simulink model "HinfDesign1_closed"  (R2018b)
settings: Solver=VariableStepAuto  StartTime=0.0  StopTime=200  RelTol=1e-3
model workspace: external: MATLAB File C:\Users\Yavuz\Documents\MATLAB\constants.m (data not in the file)
values from neighbouring files (symbols this model uses):
  alpha = 0.5736    [constants.m]
  c_damp = 0.00495    [constants.m]
  delay = 0.8    [constants.m]
  dis_torque = 0.001    [constants.m]
  in_nu = 0.0001    [constants.m]
  J_r = 0.0004    [constants.m]
  J_s = 31.38    [constants.m]
  noise = 10^-9    (= 1e-09)    [constants.m]
  T_sat = 0.05    [constants.m]
  time_cons = 0.5    [constants.m]
  w_mode = 2.6268    [constants.m]
  w_sat = 2800*2*pi/60    (= 293.215314335)    [constants.m]
libraries: cstblocks x1
settings Model: Creator=Yavuz  LastModifiedBy=Yavuz
settings DebuggingCC: AlgebraicLoopMsg=none

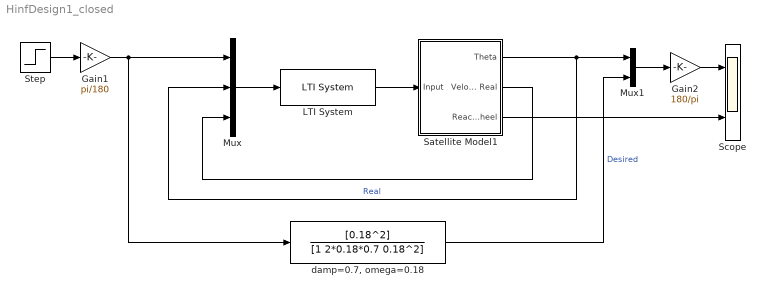
== system HinfDesign1_closed ==
  Gain1 : Gain  Gain=pi/180
  Gain2 : Gain  Gain=180/pi
  LTI System : cstblocks/LTI System  sys=K  IC=[]
  Mux : Mux  Inputs=3
  Mux1 : Mux  Inputs=2
  Satellite Model1 : Subsystem
  Scope : Scope  NumInputPorts=2
  Step : Step  Time=0  After=2.5  SampleTime=0
  "damp=0.7, omega=0.18" : TransferFcn  Numerator=[0.18^2]  Denominator=[1 2*0.18*0.7 0.18^2]
  wires:
  LTI System/1 -> Satellite Model1/1(Input)
  Gain1/1 -> Mux/1, "damp=0.7, omega=0.18"/1
  Satellite Model1/1(Theta) -> Mux/2, Mux1/1  "Real"
  Satellite Model1/2(Velocity Real) -> Mux/3
  Mux/1 -> LTI System/1
  Step/1 -> Gain1/1
  Mux1/1 -> Gain2/1
  Gain2/1 -> Scope/1
  "damp=0.7, omega=0.18"/1 -> Mux1/2  "Desired"
  Satellite Model1/3("Reaction Wheel ") -> Scope/2

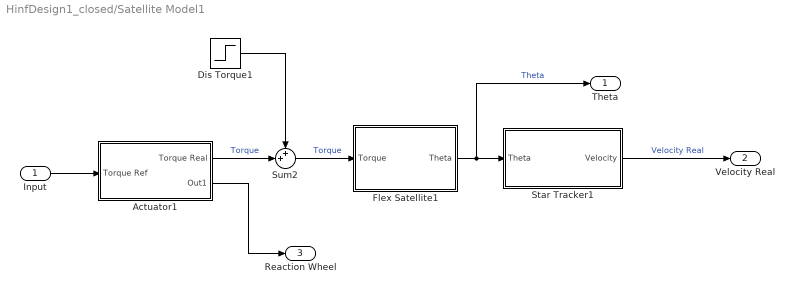
== system HinfDesign1_closed/Satellite Model1 ==
  Input : Inport
  Actuator1 : Subsystem
  Dis Torque1 : Step  Time=100  After=dis_torque  SampleTime=0
  Flex Satellite1 : Subsystem
  Star Tracker1 : Subsystem
  Sum2 : Sum  Inputs=++|
  Theta : Outport
  Velocity Real : Outport  Port=2
  "Reaction Wheel " : Outport  Port=3
  wires:
  Flex Satellite1/1(Theta) -> Star Tracker1/1(Theta), Theta/1  "Theta"
  Input/1 -> Actuator1/1(Torque Ref)
  Star Tracker1/1(Velocity) -> Velocity Real/1  "Velocity Real"
  Dis Torque1/1 -> Sum2/1
  Sum2/1 -> Flex Satellite1/1(Torque)  "Torque"
  Actuator1/1(Torque Real) -> Sum2/2  "Torque"
  Actuator1/2(Out1) -> "Reaction Wheel "/1

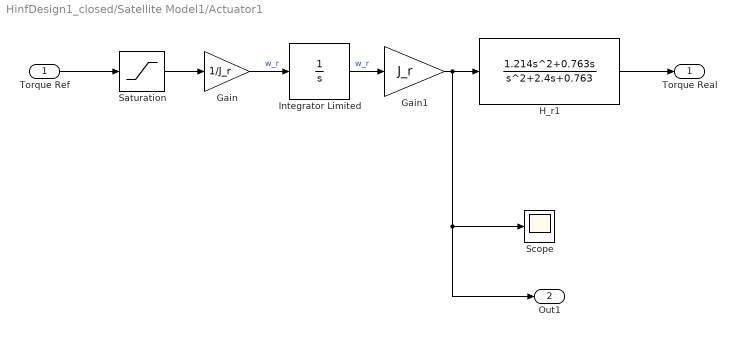
== system HinfDesign1_closed/Satellite Model1/Actuator1 ==
  Torque Ref : Inport
  Gain : Gain  Gain=1/J_r
  Gain1 : Gain  Gain=J_r
  H_r1 : TransferFcn  Numerator=[1.214 0.763 0]  Denominator=[1 2.4 0.763]
  Integrator Limited : Integrator  LimitOutput=on  UpperSaturationLimit=w_sat  LowerSaturationLimit=-w_sat
  Saturation : Saturate  UpperLimit=T_sat  LowerLimit=-T_sat
  Scope : Scope
  Torque Real : Outport
  Out1 : Outport  Port=2
  wires:
  Torque Ref/1 -> Saturation/1
  Integrator Limited/1 -> Gain1/1  "w_r"
  H_r1/1 -> Torque Real/1
  Gain1/1 -> Out1/1, Scope/1, H_r1/1
  Saturation/1 -> Gain/1
  Gain/1 -> Integrator Limited/1  "w_r"

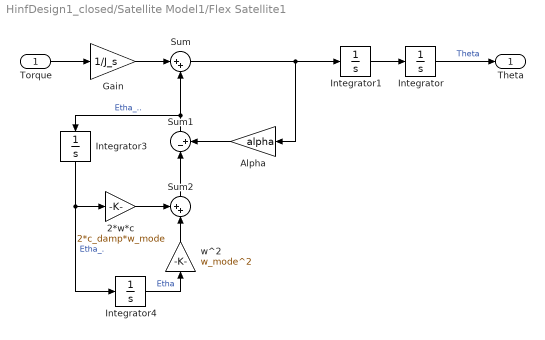
== system HinfDesign1_closed/Satellite Model1/Flex Satellite1 ==
  Torque : Inport
  2*w*c : Gain  Gain=2*c_damp*w_mode
  Alpha : Gain  Gain=alpha
  Gain : Gain  Gain=1/J_s
  Integrator : Integrator
  Integrator1 : Integrator
  Integrator3 : Integrator
  Integrator4 : Integrator  InitialCondition=in_nu
  Sum : Sum  Inputs=|++
  Sum1 : Sum  Inputs=|-+
  Sum2 : Sum  Inputs=++|
  w^2 : Gain  Gain=w_mode^2
  Theta : Outport
  wires:
  Sum/1 -> Integrator1/1, Alpha/1
  Sum1/1 -> Integrator3/1, Sum/2  "Etha_.."
  Gain/1 -> Sum/1
  Integrator1/1 -> Integrator/1
  Integrator3/1 -> Integrator4/1, 2*w*c/1  "Etha_."
  Sum2/1 -> Sum1/1
  Torque/1 -> Gain/1
  2*w*c/1 -> Sum2/1
  Integrator/1 -> Theta/1  "Theta"
  w^2/1 -> Sum2/2
  Integrator4/1 -> w^2/1  "Etha"
  Alpha/1 -> Sum1/2

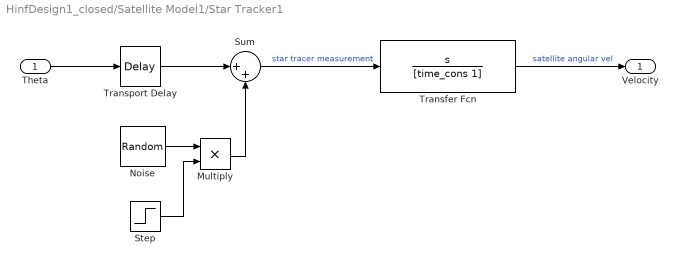
== system HinfDesign1_closed/Satellite Model1/Star Tracker1 ==
  Theta : Inport
  Multiply : Product
  Noise : RandomNumber  Variance=noise  SampleTime=0.1
  Step : Step  Time=160  SampleTime=0
  Sum : Sum  Inputs=|++
  Transfer Fcn : TransferFcn  Numerator=[1 0]  Denominator=[time_cons 1]
  Transport Delay : TransportDelay  DelayTime=delay
  Velocity : Outport
  wires:
  Transfer Fcn/1 -> Velocity/1  "satellite angular vel"
  Multiply/1 -> Sum/2
  Transport Delay/1 -> Sum/1
  Step/1 -> Multiply/2
  Theta/1 -> Transport Delay/1
  Noise/1 -> Multiply/1
  Sum/1 -> Transfer Fcn/1  "star tracer measurement"
